simulink library "scars_library"  (R2019b)
settings: Solver=VariableStepAuto  StartTime=0.0  StopTime=10.0  RelTol=1e-3
values from neighbouring files (symbols this model uses):
  startTime = 0    [SCARSSetup.m]    (also in pwsat2_setup.m; scars_setup.m)
undefined symbols (not defined in the file or in its folder): added_noise, multiplied_noise, thruster
settings Model: Creator=asmialek  LastModifiedBy=asmialek

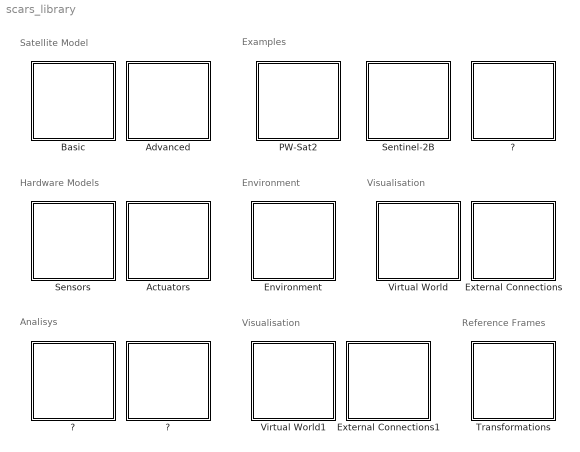
== system scars_library ==
  note: Environment
  note: Hardware Models
  note: Visualisation
  note: Examples
  note: Analisys
  note: Satellite Model
  note: Visualisation
  note: Reference Frames
  "  ?  " : Subsystem
  " ? " : Subsystem
  "?" : Subsystem
  Actuators : Subsystem
  Advanced : Subsystem
  Basic : Subsystem
  Environment : Subsystem
  External Connections : Subsystem
  External Connections1 : Subsystem
  PW-Sat2 : Subsystem
  Sensors : Subsystem
  Sentinel-2B : Subsystem
  Transformations : Subsystem
  Virtual World : Subsystem
  Virtual World1 : Subsystem

== system scars_library/  ?   ==

== system scars_library/ ?  ==

== system scars_library/? ==

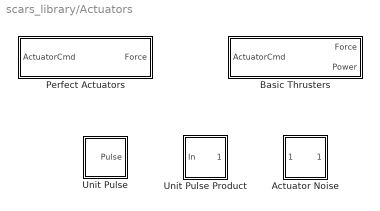
== system scars_library/Actuators ==
  Actuator Noise : Subsystem
  Basic Thrusters : Subsystem
  Perfect Actuators : Subsystem
  Unit Pulse : Subsystem
  Unit Pulse Product : Subsystem

== system scars_library/Advanced ==

== system scars_library/Basic ==

== system scars_library/Environment ==

== system scars_library/External Connections ==

== system scars_library/External Connections1 ==

== system scars_library/PW-Sat2 ==

== system scars_library/Sensors ==

== system scars_library/Sentinel-2B ==

== system scars_library/Transformations ==

== system scars_library/Virtual World ==

== system scars_library/Virtual World1 ==

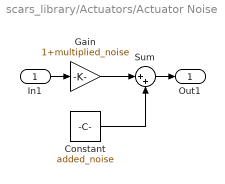
== system scars_library/Actuators/Actuator Noise ==
  In1 : Inport
  Constant : Constant  Value=added_noise
  Gain : Gain  Gain=1+multiplied_noise
  Sum : Sum  Inputs=|++
  Out1 : Outport
  wires:
  Sum/1 -> Out1/1
  In1/1 -> Gain/1
  Constant/1 -> Sum/2
  Gain/1 -> Sum/1

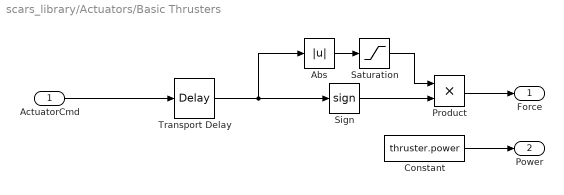
== system scars_library/Actuators/Basic Thrusters ==
  ActuatorCmd : Inport
  Abs : Abs
  Constant : Constant  Value=thruster.power
  Product : Product
  Saturation : Saturate  UpperLimit=thruster.max  LowerLimit=thruster.min
  Sign : Signum
  Transport Delay : TransportDelay  DelayTime=thruster.delay
  Force : Outport
  Power : Outport  Port=2
  wires:
  Abs/1 -> Saturation/1
  Sign/1 -> Product/2
  Saturation/1 -> Product/1
  Product/1 -> Force/1
  Transport Delay/1 -> Sign/1, Abs/1
  Constant/1 -> Power/1
  ActuatorCmd/1 -> Transport Delay/1

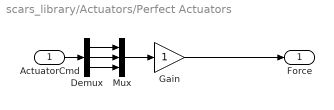
== system scars_library/Actuators/Perfect Actuators ==
  ActuatorCmd : Inport
  Demux : Demux  Outputs=3
  Gain : Gain
  Mux : Mux  Inputs=3
  Force : Outport
  wires:
  Demux/3 -> Mux/3
  Mux/1 -> Gain/1
  Demux/1 -> Mux/1
  ActuatorCmd/1 -> Demux/1
  Demux/2 -> Mux/2
  Gain/1 -> Force/1

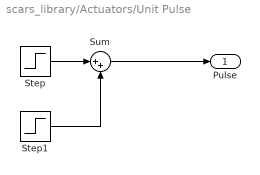
== system scars_library/Actuators/Unit Pulse ==
  Step : Step  Time=startTime  SampleTime=0
  Step1 : Step  Time=startTime+length  After=-1  SampleTime=0
  Sum : Sum  Inputs=|++
  " Pulse" : Outport
  wires:
  Sum/1 -> " Pulse"/1
  Step1/1 -> Sum/2
  Step/1 -> Sum/1

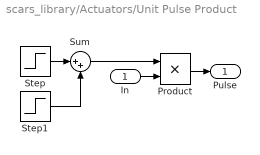
== system scars_library/Actuators/Unit Pulse Product ==
  In : Inport
  Product : Product
  Step : Step  Time=startTime  SampleTime=0
  Step1 : Step  Time=startTime+length  After=-1  SampleTime=0
  Sum : Sum  Inputs=|++
  " Pulse" : Outport
  wires:
  Step/1 -> Sum/1
  Sum/1 -> Product/1
  Step1/1 -> Sum/2
  In/1 -> Product/2
  Product/1 -> " Pulse"/1
